simulink model "stable3d"  (R2022a)
settings: Solver=FixedStepAuto  StartTime=0.0  StopTime=10  FixedStep=0.005  RelTol=1e-3
values from neighbouring files (symbols this model uses):
  x0 = 5.5 + X0(i,1)    [gen_data.m]
  y0 = -5.5 - X0(i,2)    [gen_data.m]
  z0 = 3.1 + X0(i,3)    [gen_data.m]
settings Model: Creator=diego  LastModifiedBy=diego

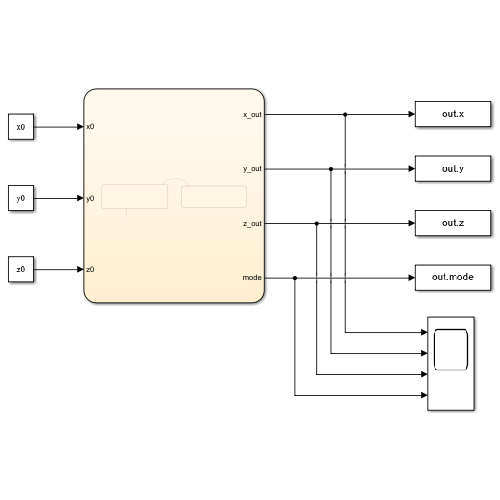
[thumbnail: Simulink's stored preview of the top-level diagram]
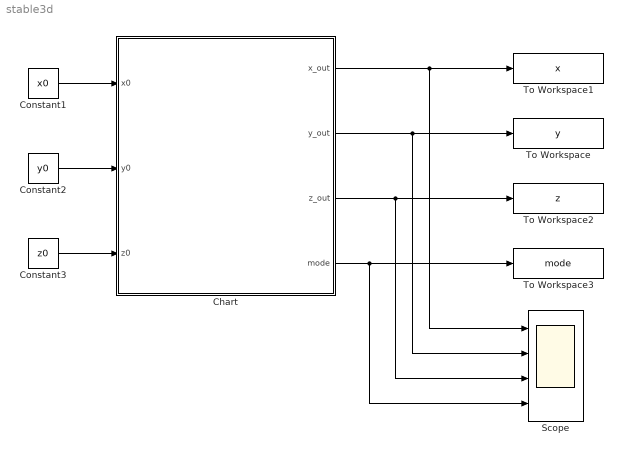
== system stable3d ==
  Chart : Stateflow chart  TreatAsAtomicUnit=on
  Constant1 : Constant  Value=x0
  Constant2 : Constant  Value=y0
  Constant3 : Constant  Value=z0
  Scope : Scope  NumInputPorts=4
  To Workspace : ToWorkspace  VariableName=y  SampleTime=-1
  To Workspace1 : ToWorkspace  VariableName=x  SampleTime=-1
  To Workspace2 : ToWorkspace  VariableName=z  SampleTime=-1
  To Workspace3 : ToWorkspace  VariableName=mode  SampleTime=-1
  wires:
  Chart/1(x_out) -> Scope/1, To Workspace1/1
  Chart/2(y_out) -> Scope/2, To Workspace/1
  Constant1/1 -> Chart/1(x0)
  Constant2/1 -> Chart/2(y0)
  Chart/3(z_out) -> Scope/3, To Workspace2/1
  Constant3/1 -> Chart/3(z0)
  Chart/4(mode) -> Scope/4, To Workspace3/1

== stateflow chart stable3d/Chart ==
  settings: updateMethod=CONTINUOUS
  state Mode1
    du:
    x_dot = -9*(x-2) -7*(y+2) + z-1 + 0.2*(x-2)*(y+2) + 0.1*(y+2)*(z-1) + 0.1*(x-2)*(z-1)+0.5*(z-1)^2;
    y_dot = 6*(x-2) + 4*(y+2) + z-1;
    z_dot = 3*(x-2) + 2*(y+2) - 2.5*(z-1);
    x_out = x;
    y_out = y;
    z_out = z;
    mode = 1;
  state Mode2
    du:
    x_dot = 2.2*x + 3.6*y + 3.9*z;
    y_dot = 3*x + 2.4*y + 3.4*z -0.01*x^2;
    z_dot = -5*x -5.4*y -6.7*z;
    x_out = x;
    y_out = y;
    z_out = z;
    mode = 2;
  Mode1 -> Mode2 : [x > 1.7 & x < 2.3 & y > -2.3 & y < -1.7 & z > 0.7 & z < 1.3]
  (default) -> Mode1 : {x = x0;
      | y = y0;
      | z = z0;}
  data: x_out output; y_out output; x local; y local; x0 input; y0 input; z_out output; z0 input; mode output; z local
  data x settings: updateMethod=SF_CONTINUOUS_TIME_DATA
  data y settings: updateMethod=SF_CONTINUOUS_TIME_DATA
  data z settings: updateMethod=SF_CONTINUOUS_TIME_DATA
